simulink model "Velo_BF"  (R2018a)
settings: Solver=ode15s  StartTime=0.0  StopTime=7  RelTol=1e-1  AbsTol=1e-3
undefined symbols (not defined in the file): AngleInitial, Kd_v, Ki_v, Kp_v
settings Model: Creator=chsira  LastModifiedBy=charl
settings DebuggingCC: AlgebraicLoopMsg=none  LibraryContextMissingDiagnostic=warning
settings ModelReferenceCC: ModelReferenceMinAlgLoopOccurrences=on
settings SFSimCC: SimUseLocalCustomCode=on
settings RTWCC: RTWUseLocalCustomCode=on

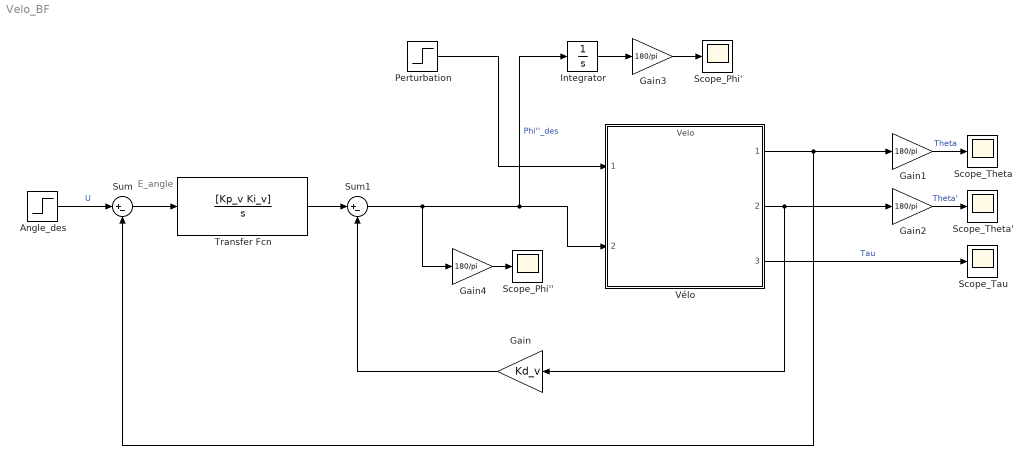
== system Velo_BF ==
  note: E_angle
  "Angle_des " : Step  Time=0  After=0*pi/180  SampleTime=0
  Gain : Gain  Gain=Kd_v
  Gain{1..4} (4 alike) : Gain  Gain=180/pi
  Integrator : Integrator
  Perturbation : Step  Time=5  After=0.05*0  SampleTime=0
  Scope_Phi' : Scope
  "Scope_Phi'' " : Scope
  Scope_Tau : Scope
  Scope_Theta : Scope
  Scope_Theta' : Scope
  Sum : Sum  Inputs=|+-
  Sum1 : Sum  Inputs=|+-
  Transfer Fcn : TransferFcn  Numerator=[Kp_v Ki_v]  Denominator=[1 0]
  Vélo : ModelReference  ModelNameDialog=Velo.slx  ParameterArgumentNames=InitialCondition  ParameterArgumentValues=InitialCondition  UsingDefaultArgumentValue=0  SimulationMode=Normal  ModelReferenceVersion=1.73  InitialCondition=AngleInitial*pi/180  SimulationMode=Normal
  wires:
  Vélo/1 -> Gain1/1, Sum/2
  "Angle_des "/1 -> Sum/1  "U"
  Gain/1 -> Sum1/2
  Sum/1 -> Transfer Fcn/1
  Sum1/1 -> Integrator/1, Vélo/2, Gain4/1  "Phi''_des"
  Transfer Fcn/1 -> Sum1/1
  Vélo/3 -> Scope_Tau/1  "Tau"
  Vélo/2 -> Gain2/1, Gain/1
  Gain1/1 -> Scope_Theta/1  "Theta"
  Gain2/1 -> Scope_Theta'/1  "Theta'"
  Integrator/1 -> Gain3/1
  Gain3/1 -> Scope_Phi'/1
  Gain4/1 -> "Scope_Phi'' "/1
  Perturbation/1 -> Vélo/1
